simulink model "pid_simulation"  (R2022b)
settings: Solver=FixedStepDiscrete  StartTime=0.0  StopTime=300  FixedStep=0.01  RelTol=1e-3
model workspace (MAT data in the model file):
  BASE_LENGTH = 0.1
libraries: mobileRoboticsTrainingLib x9, dspbuff3 x2, simulink x1, dspswit3 x1, slpidlib x1
settings Model: NumberOfSteps=100  PacingRate=0.500000  Creator=Amin Fadel  LastModifiedBy=Amin Fadel

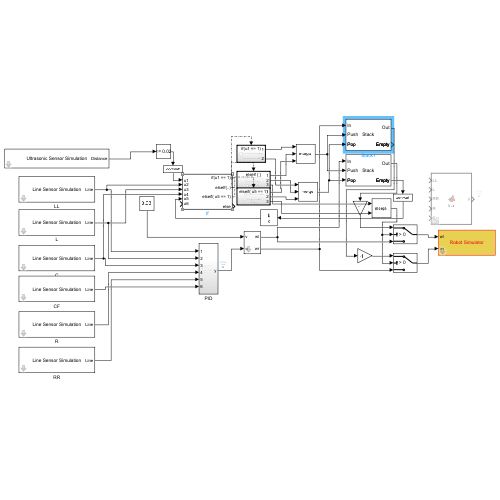
[thumbnail: Simulink's stored preview of the top-level diagram]
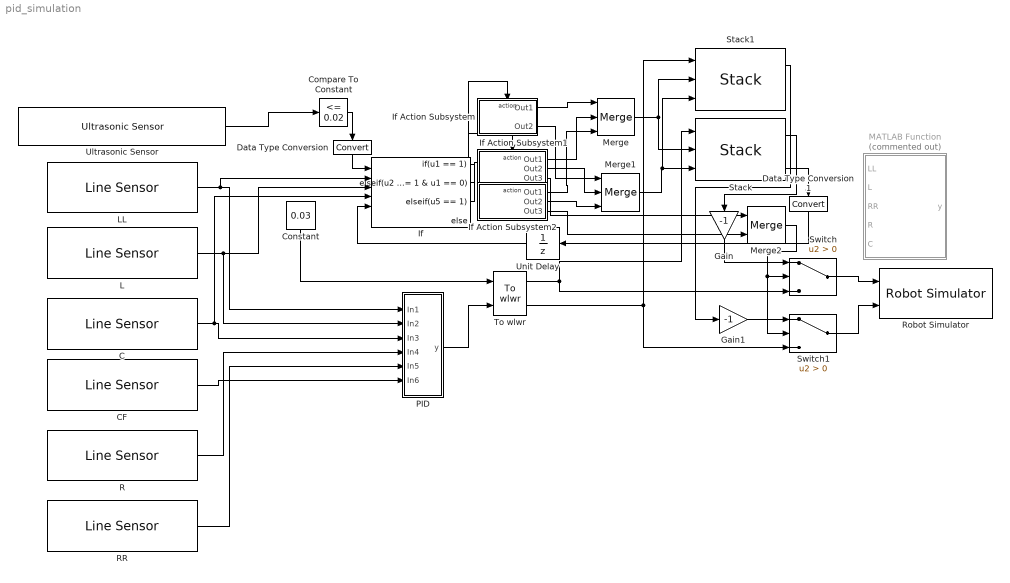
== system pid_simulation ==
  C : mobileRoboticsTrainingLib/Line Sensor  mapVariable=mapForSim  envVal=0  lineVal=1  sensOff=[BASE_LENGTH 0]
      settings: SourceProductName=Mobile Robotics Training Library
  CF : mobileRoboticsTrainingLib/Line Sensor  mapVariable=mapForSim  envVal=0  lineVal=1  sensOff=[BASE_LENGTH+0.02 0]
      settings: SourceProductName=Mobile Robotics Training Library
  Compare To Constant : simulink/Logic and Bit Operations/Compare To Constant  relop=<=  const=0.02  OutDataTypeStr=boolean
  Constant : Constant  Value=0.03
  Data Type Conversion : DataTypeConversion  SaturateOnIntegerOverflow=off  RndMeth=Floor
  Data Type Conversion1 : DataTypeConversion  SaturateOnIntegerOverflow=off  RndMeth=Floor
  Gain : Gain  Gain=-1
  Gain1 : Gain  Gain=-1
  If : If  NumInputs=6  IfExpression=u1 == 1  ElseIfExpressions=u2 == 1 & u3 == 1 & u4 == 1 & u1 == 0, u5 == 1
  If Action Subsystem : Subsystem  TreatAsAtomicUnit=on
  If Action Subsystem1 : Subsystem  TreatAsAtomicUnit=on
  If Action Subsystem2 : Subsystem  TreatAsAtomicUnit=on
  L : mobileRoboticsTrainingLib/Line Sensor  mapVariable=mapForSim  envVal=0  lineVal=1  sensOff=[BASE_LENGTH 0.04]
      settings: SourceProductName=Mobile Robotics Training Library
  LL : mobileRoboticsTrainingLib/Line Sensor  mapVariable=mapForSim  envVal=0  lineVal=1  sensOff=[BASE_LENGTH 0.1]
      settings: SourceProductName=Mobile Robotics Training Library
  MATLAB Function : MATLAB Function  Commented=on  TreatAsAtomicUnit=on
  Merge : Merge  Inputs=3
  Merge1 : Merge  Inputs=3
  Merge2 : Merge
  PID : Subsystem
  R : mobileRoboticsTrainingLib/Line Sensor  mapVariable=mapForSim  envVal=0  lineVal=1  sensOff=[BASE_LENGTH -0.04]
      settings: SourceProductName=Mobile Robotics Training Library
  RR : mobileRoboticsTrainingLib/Line Sensor  mapVariable=mapForSim  envVal=0  lineVal=1  sensOff=[BASE_LENGTH -0.1]
      settings: SourceProductName=Mobile Robotics Training Library
  Robot Simulator : mobileRoboticsTrainingLib/Robot Simulator  Priority=99  mapVar=mapForSim  startX=1.41107871720117  startY=1.44314868804665  startTheta=-90  axleLength=0.1  wheelR=0.05
  Stack : dspbuff3/Stack  depth=16000  trigger=Non-zero sample  overflow=Dynamic reallocation  pes=Warning  eso=on  fso=off  nso=off  clr=off  clrOutport=off
  Stack1 : dspbuff3/Stack  depth=16000  trigger=Non-zero sample  overflow=Dynamic reallocation  pes=Warning  eso=on  fso=off  nso=off  clr=off  clrOutport=off
  Switch : Switch  Criteria=u2 > Threshold  SaturateOnIntegerOverflow=off  InputSameDT=off
  Switch1 : Switch  Criteria=u2 > Threshold  SaturateOnIntegerOverflow=off  InputSameDT=off
  To wlwr : mobileRoboticsTrainingLib/To wlwr  axleLength=0.1  wheelR=0.05
  Ultrasonic Sensor : mobileRoboticsTrainingLib/Ultrasonic Sensor  mapVar=mapForSim  maxSenRange=2  minSenRange=0.01  senRes=0.01  sensOff=[BASE_LENGTH 0]
      settings: SourceProductName=Mobile Robotics Training Library
  Unit Delay : UnitDelay  SampleTime=-1  HasFrameUpgradeWarning=on
  wires:
  To wlwr/1 -> Stack/1, Switch/3
  To wlwr/2 -> Switch1/3, Stack1/1
  Constant/1 -> To wlwr/1
  PID/1(y) -> To wlwr/2
  LL/1 -> If/2, PID/1(In1)
  L/1 -> If/3, PID/2(In2)
  C/1 -> If/4, PID/3(In3)
  CF/1 -> PID/6(In6)
  RR/1 -> PID/5(In5)
  R/1 -> PID/4(In4)
  Ultrasonic Sensor/1 -> Compare To Constant/1
  Compare To Constant/1 -> Data Type Conversion/1
  If/1 -> If Action Subsystem/Action
  If/2 -> If Action Subsystem1/Action
  If Action Subsystem/1(Out1) -> Merge/1
  If Action Subsystem1/1(Out1) -> Merge/2
  Merge/1 -> Stack/2, Stack1/2
  If Action Subsystem1/2(Out2) -> Merge1/2
  If Action Subsystem/2(Out2) -> Merge1/1
  Merge1/1 -> Stack1/3, Stack/3
  Stack/2 -> Data Type Conversion1/1
  Unit Delay/1 -> If/5
  If/3 -> If Action Subsystem2/Action
  If Action Subsystem2/2(Out2) -> Merge1/3
  If Action Subsystem2/1(Out1) -> Merge/3
  If Action Subsystem1/3(Out3) -> Merge2/1
  If Action Subsystem2/3(Out3) -> Merge2/2
  Merge2/1 -> Switch1/2, Switch/2
  Stack/1 -> Gain/1
  Switch/1 -> Robot Simulator/1
  Data Type Conversion/1 -> If/1
  Data Type Conversion1/1 -> Unit Delay/1
  Gain/1 -> Switch/1
  Stack1/1 -> Gain1/1
  Gain1/1 -> Switch1/1
  Switch1/1 -> Robot Simulator/2

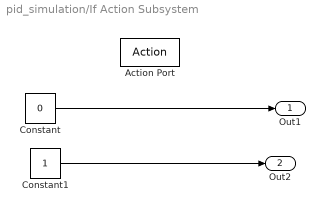
== system pid_simulation/If Action Subsystem ==
  Action Port : ActionPort  ActionPortLabel=if(u1 == 1)
  Constant : Constant  Value=0
  Constant1 : Constant
  Out1 : Outport
  Out2 : Outport  Port=2
  wires:
  Constant/1 -> Out1/1
  Constant1/1 -> Out2/1

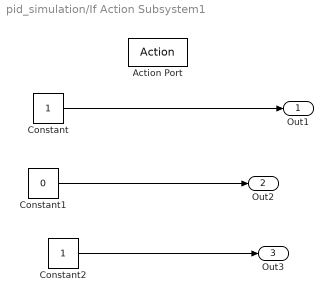
== system pid_simulation/If Action Subsystem1 ==
  Action Port : ActionPort  ActionPortLabel=elseif(u2 == 1 & u3 == 1 & u4 == 1 & u1 == 0)
  Constant : Constant
  Constant1 : Constant  Value=0
  Constant2 : Constant
  Out1 : Outport
  Out2 : Outport  Port=2
  Out3 : Outport  Port=3
  wires:
  Constant/1 -> Out1/1
  Constant1/1 -> Out2/1
  Constant2/1 -> Out3/1

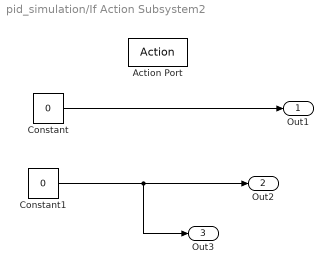
== system pid_simulation/If Action Subsystem2 ==
  Action Port : ActionPort  ActionPortLabel=elseif( u5 == 1)
  Constant : Constant  Value=0
  Constant1 : Constant  Value=0
  Out1 : Outport
  Out2 : Outport  Port=2
  Out3 : Outport  Port=3
  wires:
  Constant/1 -> Out1/1
  Constant1/1 -> Out3/1, Out2/1

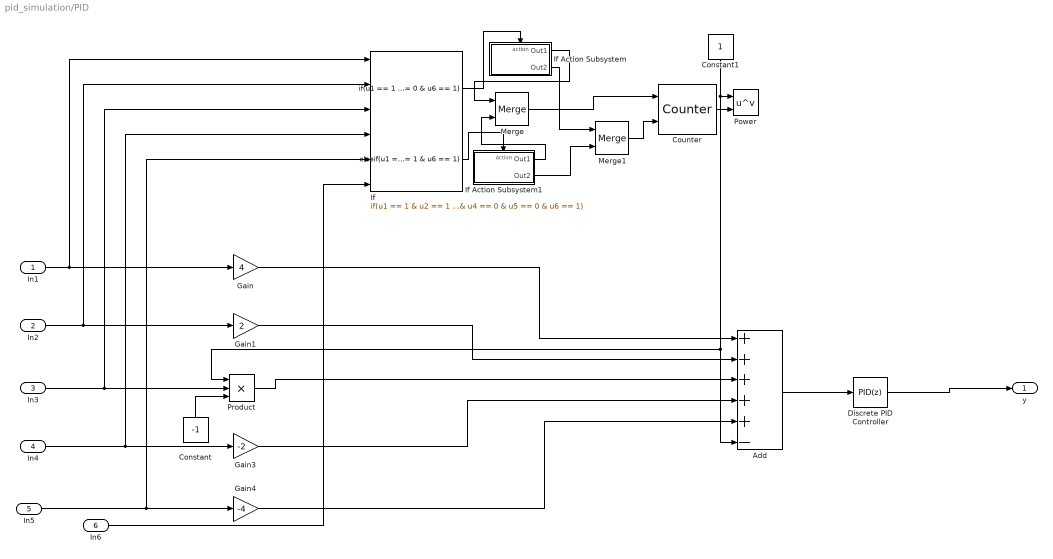
== system pid_simulation/PID ==
  In1 : Inport
  In2 : Inport  Port=2
  In3 : Inport  Port=3
  In4 : Inport  Port=4
  In5 : Inport  Port=5
  In6 : Inport  Port=6
  Add : Sum  Inputs=+++++-
  Constant : Constant  Value=-1
  Constant1 : Constant
  Counter : dspswit3/Counter  Direction=Up  CountEvent=Non-zero sample  CounterSize=User defined  MaxCount=1  InitialCount=0  Output=Count  HitValue=32  ResetInput=on  SamplesPerFrame=1  Ts=1  CntDtype=double  HitDtype=Logical
  Discrete PID Controller : slpidlib/PID Controller  Controller=PID  Form=Parallel  TimeDomain=Discrete-time  UseExternalTs=off  SampleTime=-1  IntegratorMethod=Forward Euler  FilterMethod=Forward Euler  ControllerParametersSource=internal  P=1  I=10  UseKiTs=off  D=0  N=100  UseFilter=on  TunerSelectOption=Frequency Response Based  InitialConditionSource=internal  InitialConditionForIntegrator=0  InitialConditionForFilter=0  DifferentiatorICPrevScaledInput=0  ExternalReset=none  TrackingMode=off  Kt=1  LimitOutput=off  SatLimitsSource=internal  UpperSaturationLimit=inf  LowerSaturationLimit=-inf  LinearizeAsGain=off  AntiWindupMode=none  Kb=1  LimitIntegrator=off  UpperIntegratorSaturationLimit=inf  LowerIntegratorSaturationLimit=-inf  POutMin=[]  POutMax=[]  IOutMin=[]  IOutMax=[]  DOutMin=[]  DOutMax=[]  NOutMin=[]  NOutMax=[]  SumOutMin=[]  SumOutMax=[]  SaturationOutMin=[]  SaturationOutMax=[]  PParamMin=[]  PParamMax=[]  IParamMin=[]  IParamMax=[]  DParamMin=[]  DParamMax=[]  NParamMin=[]  NParamMax=[]  KbParamMin=[]  KbParamMax=[]  KtParamMin=[]  KtParamMax=[]  KbOutMin=[]  KbOutMax=[]  KtOutMin=[]  KtOutMax=[]  IntegratorOutMin=[]  IntegratorOutMax=[]  FilterOutMin=[]  FilterOutMax=[]  SumI1OutMin=[]  SumI1OutMax=[]  SumI2OutMin=[]  SumI2OutMax=[]  SumI3OutMin=[]  SumI3OutMax=[]  SumI4OutMin=[]  SumI4OutMax=[]  SumDOutMin=[]  SumDOutMax=[]  DifferentiatorOutMin=[]  DifferentiatorOutMax=[]  FilterDiffOutCoefMin=[]  FilterDiffOutCoefMax=[]  ReciprocalOutMin=[]  ReciprocalOutMax=[]  SumDenOutMin=[]  SumDenOutMax=[]  SumNumOutMin=[]  SumNumOutMax=[]  DivideOutMin=[]  DivideOutMax=[]  UdiffTsProdOutMin=[]  UdiffTsProdOutMax=[]  NTsProdOutMin=[]  NTsProdOutMax=[]  UintegralTsProdOutMin=[]  UintegralTsProdOutMax=[]  UngainTsProdOutMin=[]  UngainTsProdOutMax=[]  ClampingZeroOutDataTypeStr=Inherit: Inherit via back propagation  ClampingZeroOutMin=[]  ClampingZeroOutMax=[]  FilterDenConstantOutDataTypeStr=Inherit: Inherit via back propagation  FilterDenConstantOutMin=[]  FilterDenConstantOutMax=[]  PCopyOutDataTypeStr=Inherit: Inherit via back propagation  PCopyOutMin=[]  PCopyOutMax=[]  NCopyOutDataTypeStr=Inherit: Inherit via back propagation  NCopyOutMin=[]  NCopyOutMax=[]  IntegratorContinuousStateAttributes=''  IntegratorStateMustResolveToSignalObject=off  IntegratorRTWStateStorageClass=Auto  FilterContinuousStateAttributes=''  FilterStateMustResolveToSignalObject=off  FilterRTWStateStorageClass=Auto  ParallelPVariant=InternalParameters  IdealPVariant=Disabled  IVariant=InternalParameters  DVariant=InternalParameters  IntegratorVariant=Discrete  SatVariant=Disabled  AWVariant=Passthrough  PCopyVariant=Disabled  TRVariant=Disabled  FdbkBlocksVariant=Forward  IdealPFdbkVariant=Disabled  SatFdbkVariant=Disabled  DerivativeFilterVariant=ForwardEulerFilter  NVariant=InternalParameters  NCopyVariant=Disabled  FilterICVariant=InternalICsFilter  IntegratorICVariant=InternalICs  ExternalResetVariant=Disabled  TRSumVariant=Passthrough  SumFdbkVariant=Disabled  SumVariant=Sum_PID  TsampFilterVariant=InternalTs  TsampNgainVariant=Passthrough  TsampIntegralVariant=Passthrough  ExternalSaturationOutDataTypeStr=Inherit: Same as second input
      settings: LibrarySourceBlock=simulink/Discrete/Discrete PID Controller
  Gain : Gain  Gain=4
  Gain1 : Gain  Gain=2
  Gain3 : Gain  Gain=-2
  Gain4 : Gain  Gain=-4
  If : If  NumInputs=6  IfExpression=u1 == 1 & u2 == 1 & u3 == 1 & u4 == 0 & u5 == 0 & u6 == 1  ElseIfExpressions=u1 == 0 & u2 == 0 & u3 == 1 & u4 == 1 & u5 == 1 & u6 == 1  ShowElse=off
  If Action Subsystem : Subsystem  TreatAsAtomicUnit=on
  If Action Subsystem1 : Subsystem  TreatAsAtomicUnit=on
  Merge : Merge
  Merge1 : Merge
  Power : Math  Operator=pow
  Product : Product  Inputs=3
  y : Outport
  wires:
  Gain1/1 -> Add/2
  Gain/1 -> Add/1
  Product/1 -> Add/3
  In4/1 -> If/4, Gain3/1
  Discrete PID Controller/1 -> y/1
  Add/1 -> Discrete PID Controller/1
  Gain4/1 -> Add/5
  Gain3/1 -> Add/4
  In1/1 -> If/1, Gain/1
  In3/1 -> Product/2, If/3
  In2/1 -> If/2, Gain1/1
  In5/1 -> If/5, Gain4/1
  Counter/1 -> Power/2
  Constant1/1 -> Product/1, Add/6, Power/1
  If/1 -> If Action Subsystem/Action
  If/2 -> If Action Subsystem1/Action
  Constant/1 -> Product/3
  In6/1 -> If/6
  If Action Subsystem/1(Out1) -> Merge/1
  If Action Subsystem1/1(Out1) -> Merge/2
  Merge/1 -> Counter/1
  If Action Subsystem1/2(Out2) -> Merge1/2
  If Action Subsystem/2(Out2) -> Merge1/1
  Merge1/1 -> Counter/2

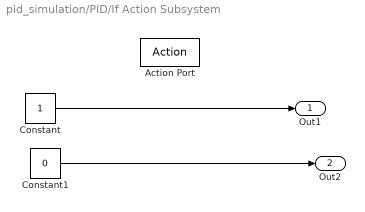
== system pid_simulation/PID/If Action Subsystem ==
  Action Port : ActionPort  ActionPortLabel=if(u1 == 1 & u2 == 1 & u3 == 1 & u4 == 0 & u5 == 0 & u6 == 1)
  Constant : Constant
  Constant1 : Constant  Value=0
  Out1 : Outport
  Out2 : Outport  Port=2
  wires:
  Constant/1 -> Out1/1
  Constant1/1 -> Out2/1

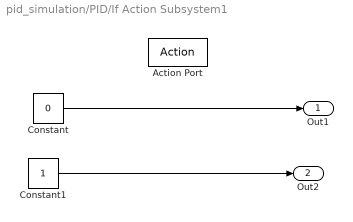
== system pid_simulation/PID/If Action Subsystem1 ==
  Action Port : ActionPort  ActionPortLabel=elseif(u1 == 0 & u2 == 0 & u3 == 1 & u4 == 1 & u5 == 1 & u6 == 1)
  Constant : Constant  Value=0
  Constant1 : Constant
  Out1 : Outport
  Out2 : Outport  Port=2
  wires:
  Constant/1 -> Out1/1
  Constant1/1 -> Out2/1

== matlab function pid_simulation/MATLAB Function ==
  data: LL input; y output; L input; RR input; R input; C input
function y = fcn(LL,L,RR,R,C)
sensorReadings =((2^4)*LL + (2^3)*L + (2^2)*RR + (2^1)*R + (2^0)*C)/100;
trajectory = [0 -5 -20 5 20];
firstHighBit = 1;
for i=5:-1:1
        isHigh = bitget(sensorReadings,i);
        if (isHigh == 1)
            firstHighBit = i;
            break
        end
end

y = trajectory(firstHighBit);
